simulink model "Controller"  (R2022b)
settings: Solver=FixedStepDiscrete  StartTime=0.0  StopTime=10.0  FixedStep=CONTROL_CONST.dt  MaxStep=CONTROL_PARAM.dt  RelTol=1e-3
values from neighbouring files (symbols this model uses):
  CONTROL_PARAM = Simulink.Parameter(CONTROL_PARAM_VALUE)    [controller_init.m]
undefined symbols (not defined in the file or in its folder): actuator_cmd, CONTROL_CONST, DiscIntNeverNeededParam, timestamp
libraries: drivingvehiclecontroller x2, simulink x1, FMT_Model_Lib x1
settings Model: Creator=19114  LastModifiedBy=19114
settings OptimizationCC: DefaultParameterBehavior=Inlined  DefaultUnderspecifiedDataType=single  EnhancedBackFolding=on  PassReuseOutputArgsAs=Individual arguments  ZeroExternalMemoryAtStartup=off  ZeroInternalMemoryAtStartup=off  OptimizeBlockOrder=speed  DifferentSizesBufferReuse=on  OptimizationCustomize=off  EfficientTunableParamExpr=on
settings DebuggingCC: ParameterTunabilityLossMsg=error  UnconnectedInputMsg=warning  UnconnectedOutputMsg=warning  UnconnectedLineMsg=warning
settings HardwareCC: ProdBitPerPointer=32  ProdBitPerSizeT=32  ProdBitPerPtrDiffT=32  ProdLargestAtomicInteger=Long  ProdLargestAtomicFloat=Double  ProdWordSize=32  ProdHWDeviceType=ARM Compatible->ARM Cortex-M
settings ModelReferenceCC: EnableRefExpFcnMdlSchedulingChecks=on
settings RTWCC: Description=Embedded Coder  SystemTargetFile=ert.tlc  TemplateMakefile=ert_default_tmf  DLArmComputeVersion=19.05
settings CodeAppCC: ForceParamTrailComments=on  IgnoreCustomStorageClasses=off  OperatorAnnotations=on  SimulinkDataObjDesc=on  SFDataObjDesc=on  InsertBlockDesc=on
settings ERTTargetCC: TargetLangStandard=C99 (ISO)  CodeReplacementLibrary=STM32 DSP LIB  GenerateSampleERTMain=on  SupportNonFinite=off  SupportVariableSizeSignals=on  InlinedParameterPlacement=NonHierarchical  ERTCustomFileTemplate=example_file_process.tlc

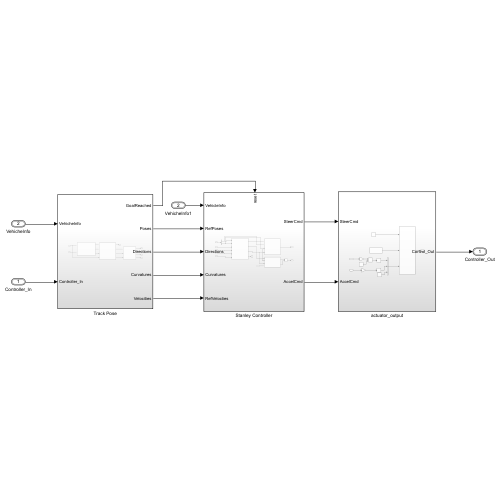
[thumbnail: Simulink's stored preview of the top-level diagram]
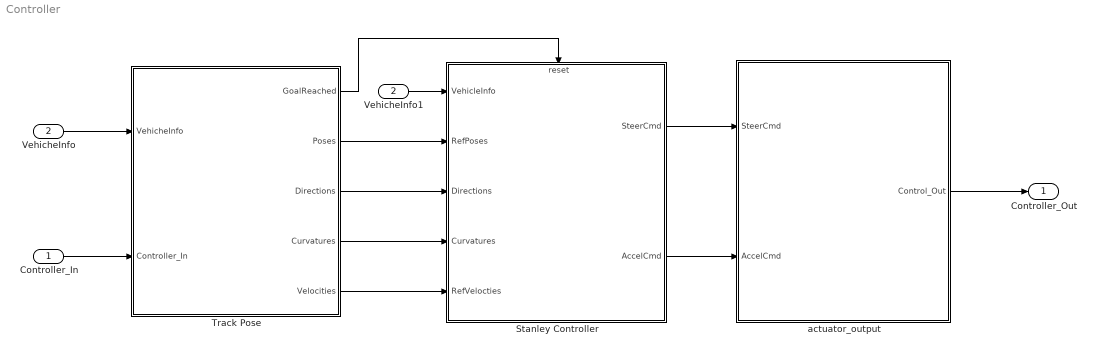
== system Controller ==
  Controller_In : Inport  OutDataTypeStr=Bus: Controller_In_Bus
  VehicheInfo : Inport  Port=2  OutDataTypeStr=Bus: VehicheInfo_Bus
  Stanley Controller : Subsystem
      settings: PortSchema="{\"entries\":[{\"content\":{\"sides\":[{\"content\":{\"connectorIds\":[\"In1\",\"In2\",\"In3\",\"In4\",\"In5\"]},\"type\":\"ConnectorPlacement.EquallySpacedRectSide\",\"uuid\":\"91070305-29de-4808-baf6-dcc08d2076f6\"},{\"content\":{\"connectorIds\":[\"Out1\",\"Out2\"],\"side\":\"RIGHT\"},\"type\":\"ConnectorPlacement.EquallySpacedRectSide\",\"uuid\":\"ca97d8aa-66c0-44c7-8bf0-9bd2dfebf383\"},{\"content\":{\"connectorIds\":[\"In6\"],\"side\":\"TOP\"},\"type\":\"ConnectorPlacement.EquallySpacedRectSide\",\"uuid\":\"0b1186ad-a9e2-4df0-8133-481be95c9fc4\"},{\"content\":{\"connectorIds\":[],\"side\":\"BOTTOM\"},\"type\":\"ConnectorPlacement.EquallySpacedRectSide\",\"uuid\":\"ab154ce3-e196-4faf-b6b9-1e885093f3b6\"}]},\"type\":\"ConnectorPlacement.EquallySpacedConnector\",\"uuid\":\"3fcf1bb3-7915-4a36-93c3-601b19fd5f1b\"}],\"packageUris\":[\"http://schema.mathworks.com/mf0/Connector/R2020b\"],\"version\":\"1.0\"}"
  Track Pose : Subsystem
  VehicheInfo1 : InportShadow  Port=2  OutDataTypeStr=Bus: VehicheInfo_Bus
  actuator_output : Subsystem
  Controller_Out : Outport  OutDataTypeStr=Bus: Controller_Out_Bus
  wires:
  Stanley Controller/1(SteerCmd) -> actuator_output/1(SteerCmd)
  Stanley Controller/2(AccelCmd) -> actuator_output/2(AccelCmd)
  actuator_output/1(Control_Out) -> Controller_Out/1
  VehicheInfo/1 -> Track Pose/1(VehicheInfo)
  Controller_In/1 -> Track Pose/2(Controller_In)
  Track Pose/1(GoalReached) -> Stanley Controller/6(reset)
  Track Pose/2(Poses) -> Stanley Controller/2(RefPoses)
  Track Pose/3(Directions) -> Stanley Controller/3(Directions)
  Track Pose/4(Curvatures) -> Stanley Controller/4(Curvatures)
  Track Pose/5(Velocities) -> Stanley Controller/5(RefVelocties)
  VehicheInfo1/1 -> Stanley Controller/1(VehicleInfo)

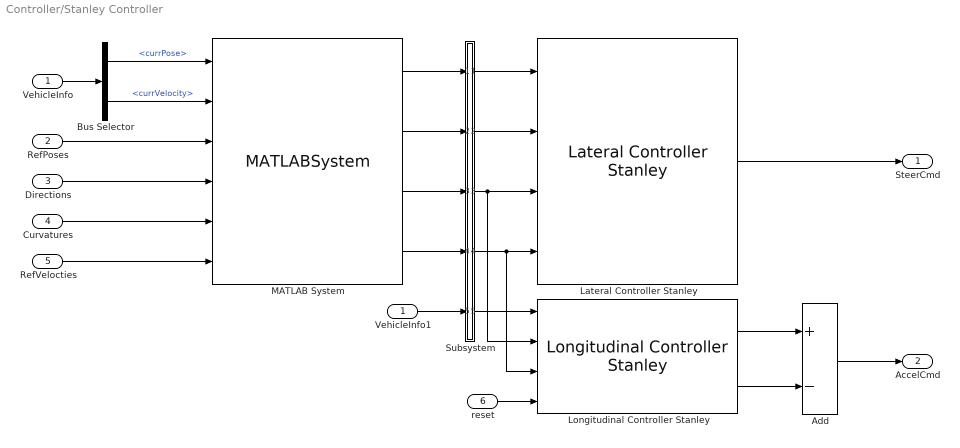
== system Controller/Stanley Controller ==
  VehicleInfo : Inport
  RefPoses : Inport  Port=2
  Directions : Inport  Port=3
  Curvatures : Inport  Port=4
  RefVelocties : Inport  Port=5
  reset : Inport  Port=6
  Add : Sum  Inputs=+-
  Bus Selector : BusSelector  OutputSignals=currPose,currVelocity
  Lateral Controller Stanley : drivingvehiclecontroller/Lateral Controller Stanley  ModelType=Kinematic bicycle model  PositionGainF=2  PositionGainR=2.5  YawRateGain=0.25  DelayGain=0.2  VehicleMass=5  Lf=1.2  Lr=1.6  TireStiffness=19e3  Wheelbase=0.3  MaxSteeringAngle=30
  Longitudinal Controller Stanley : drivingvehiclecontroller/Longitudinal Controller Stanley  Kp=CONTROL_PARAM.KP  Ki=CONTROL_PARAM.KI  SampleTime=CONTROL_CONST.dt  MaxAcceleration=20  MaxDeceleration=20
  MATLAB System : MATLABSystem  System=HelperPathAnalyzer  Wheelbase=2.8  HasResetOutput=off  SimulateUsing=Code generation
      mask Type: HelperPathAnalyzer
      mask Display:
      | disp(['Helper' char(10) 'Path' char(10) 'Analyzer']);
      | port_label('input',1,'CurrPose');
      | port_label('input',2,'CurrVelocity');
      | port_label('input',3,'RefPoses');
      | port_label('input',4,'Directions');
      | port_label('input',5,'Curvatures');
      | port_label('input',6,'RefVelocities');
      | port_label('output',1,'RefPose');
      | port_label('output',2,'RefVelocity');
      | port_label('output',3,'Direction');
      | port_label('output',4,'Curvature');
  Subsystem : Subsystem
  VehicleInfo1 : InportShadow
  SteerCmd : Outport
  AccelCmd : Outport  Port=2
  wires:
  VehicleInfo/1 -> Bus Selector/1
  Bus Selector/2 -> MATLAB System/2  "<currVelocity>"
  Bus Selector/1 -> MATLAB System/1  "<currPose>"
  RefPoses/1 -> MATLAB System/3
  Directions/1 -> MATLAB System/4
  Curvatures/1 -> MATLAB System/5
  RefVelocties/1 -> MATLAB System/6
  Lateral Controller Stanley/1 -> SteerCmd/1
  Longitudinal Controller Stanley/1 -> Add/1
  Longitudinal Controller Stanley/2 -> Add/2
  Add/1 -> AccelCmd/1
  reset/1 -> Longitudinal Controller Stanley/4
  MATLAB System/1 -> Subsystem/1(RefPose)
  MATLAB System/2 -> Subsystem/2(RefVelocity)
  MATLAB System/3 -> Subsystem/3(Direction)
  MATLAB System/4 -> Subsystem/4(Curvature)
  VehicleInfo1/1 -> Subsystem/5(VehicleInfo)
  Subsystem/1(RefPose1) -> Lateral Controller Stanley/1
  Subsystem/2(CurrPose) -> Lateral Controller Stanley/2
  Subsystem/3(CurrVelocity) -> Longitudinal Controller Stanley/2, Lateral Controller Stanley/3
  Subsystem/4(Direction1) -> Longitudinal Controller Stanley/3, Lateral Controller Stanley/4
  Subsystem/5(RefVelocity1) -> Longitudinal Controller Stanley/1

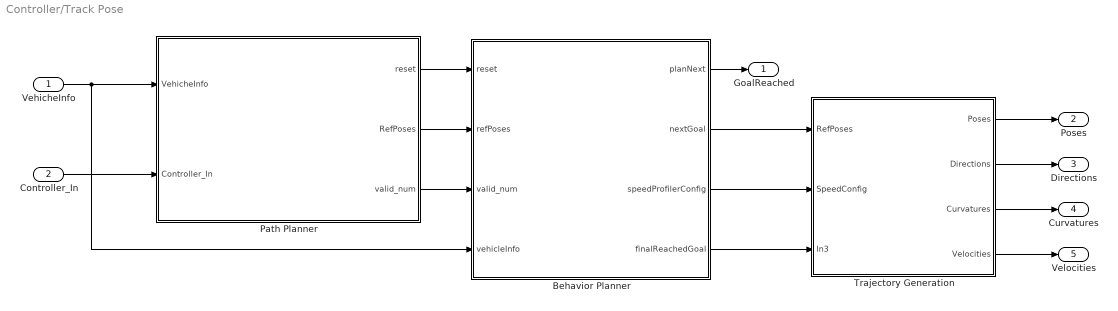
== system Controller/Track Pose ==
  VehicheInfo : Inport
  Controller_In : Inport  Port=2
  Behavior Planner : MATLAB Function  TreatAsAtomicUnit=on
  Path Planner : Subsystem
  Trajectory Generation : Subsystem
  GoalReached : Outport
  Poses : Outport  Port=2
  Directions : Outport  Port=3
  Curvatures : Outport  Port=4
  Velocities : Outport  Port=5
  wires:
  Behavior Planner/4(finalReachedGoal) -> Trajectory Generation/3(In3)
  Behavior Planner/3(speedProfilerConfig) -> Trajectory Generation/2(SpeedConfig)
  Trajectory Generation/2(Directions) -> Directions/1
  Path Planner/1(reset) -> Behavior Planner/1(reset)
  Path Planner/3(valid_num) -> Behavior Planner/3(valid_num)
  Behavior Planner/2(nextGoal) -> Trajectory Generation/1(RefPoses)
  Path Planner/2(RefPoses) -> Behavior Planner/2(refPoses)
  Trajectory Generation/3(Curvatures) -> Curvatures/1
  Behavior Planner/1(planNext) -> GoalReached/1
  VehicheInfo/1 -> Behavior Planner/4(vehicleInfo), Path Planner/1(VehicheInfo)
  Trajectory Generation/4(Velocities) -> Velocities/1
  Trajectory Generation/1(Poses) -> Poses/1
  Controller_In/1 -> Path Planner/2(Controller_In)

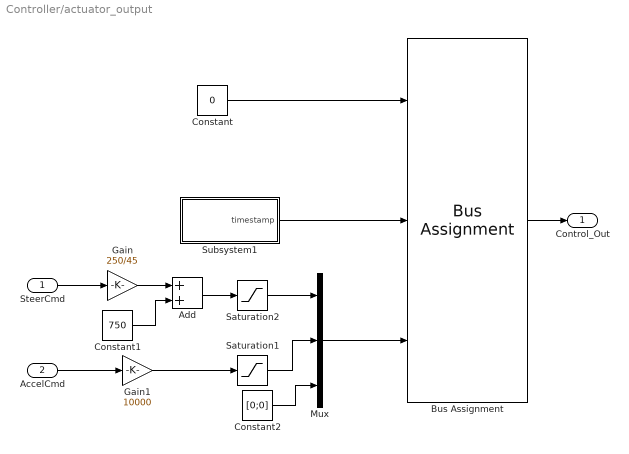
== system Controller/actuator_output ==
  SteerCmd : Inport
  AccelCmd : Inport  Port=2
  Add : Sum
  Bus Assignment : BusAssignment  AssignedSignals=timestamp,actuator_cmd
  Constant : Constant  Value=0  OutDataTypeStr=Bus: Controller_Out_Bus
  Constant1 : Constant  Value=750
  Constant2 : Constant  Value=[0;0]  OutDataTypeStr=int16
  Gain : Gain  Gain=250/45
  Gain1 : Gain  Gain=10000
  Mux : Mux  Inputs=3
  Saturation1 : Saturate  UpperLimit=10000  LowerLimit=-10000  OutDataTypeStr=int16
  Saturation2 : Saturate  UpperLimit=1250  LowerLimit=250  OutDataTypeStr=int16
  Subsystem1 : Subsystem
  Control_Out : Outport
  wires:
  Saturation2/1 -> Mux/1
  SteerCmd/1 -> Gain/1
  Saturation1/1 -> Mux/2
  Gain1/1 -> Saturation1/1
  Subsystem1/1(timestamp) -> Bus Assignment/2
  Mux/1 -> Bus Assignment/3
  Constant2/1 -> Mux/3
  Constant1/1 -> Add/2
  Add/1 -> Saturation2/1
  Constant/1 -> Bus Assignment/1
  Gain/1 -> Add/1
  Bus Assignment/1 -> Control_Out/1
  AccelCmd/1 -> Gain1/1

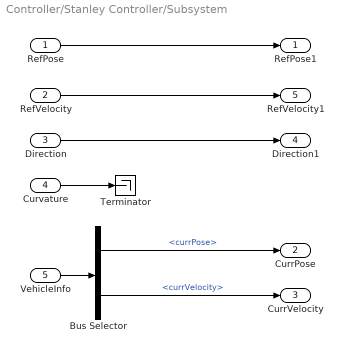
== system Controller/Stanley Controller/Subsystem ==
  RefPose : Inport
  RefVelocity : Inport  Port=2
  Direction : Inport  Port=3
  Curvature : Inport  Port=4
  VehicleInfo : Inport  Port=5
  Bus Selector : BusSelector  OutputSignals=currPose,currVelocity
  Terminator : Terminator
  RefPose1 : Outport
  CurrPose : Outport  Port=2
  CurrVelocity : Outport  Port=3
  Direction1 : Outport  Port=4
  RefVelocity1 : Outport  Port=5
  wires:
  RefPose/1 -> RefPose1/1
  VehicleInfo/1 -> Bus Selector/1
  Bus Selector/1 -> CurrPose/1  "<currPose>"
  Bus Selector/2 -> CurrVelocity/1  "<currVelocity>"
  Direction/1 -> Direction1/1
  RefVelocity/1 -> RefVelocity1/1
  Curvature/1 -> Terminator/1

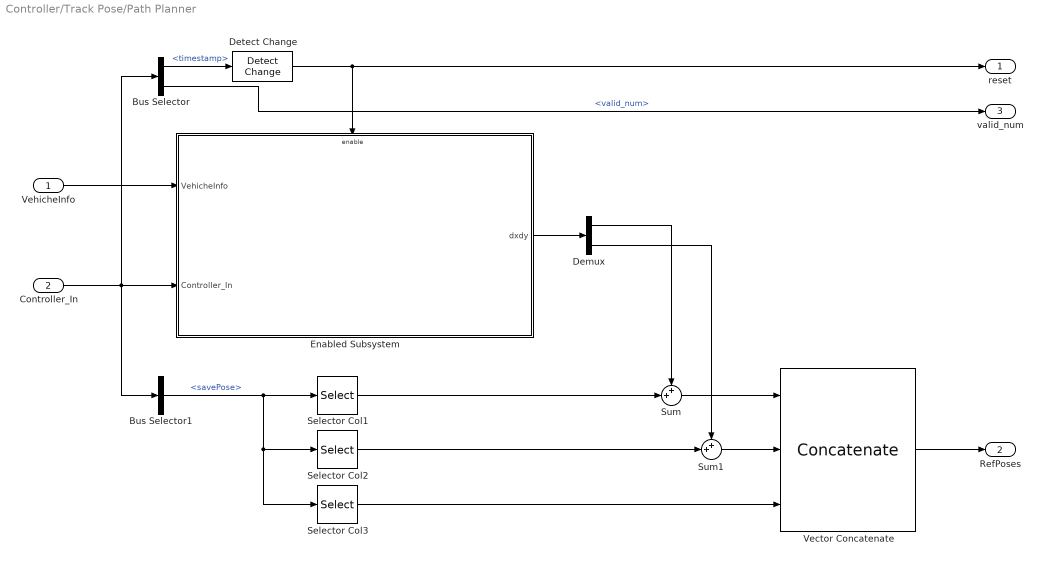
== system Controller/Track Pose/Path Planner ==
  VehicheInfo : Inport
  Controller_In : Inport  Port=2
  Bus Selector : BusSelector  OutputSignals=timestamp,valid_num
  Bus Selector1 : BusSelector  OutputSignals=savePose
  Demux : Demux  Outputs=2
  Detect Change : simulink/Logic and Bit Operations/Detect Change  vinit=0  OutDataTypeStr=boolean
  Enabled Subsystem : Subsystem  TreatAsAtomicUnit=on
  Selector Col1 : Selector  NumberOfDimensions=2  InputPortWidth=3  IndexOptions=Select all,Index vector (dialog)  Indices=[1 3],1  OutputSizes=1,1
  Selector Col2 : Selector  NumberOfDimensions=2  InputPortWidth=3  IndexOptions=Select all,Index vector (dialog)  Indices=[1 3],2  OutputSizes=1,1
  Selector Col3 : Selector  NumberOfDimensions=2  InputPortWidth=3  IndexOptions=Select all,Index vector (dialog)  Indices=[1 3],3  OutputSizes=1,1
  Sum : Sum  Inputs=++|
  Sum1 : Sum  Inputs=++|
  Vector Concatenate : Concatenate  NumInputs=3  Mode=Multidimensional array  ConcatenateDimension=2
  reset : Outport
  RefPoses : Outport  Port=2
  valid_num : Outport  Port=3
  wires:
  Bus Selector/1 -> Detect Change/1  "<timestamp>"
  Bus Selector1/1 -> Selector Col3/1, Selector Col2/1, Selector Col1/1  "<savePose>"
  Selector Col1/1 -> Sum/2
  Demux/2 -> Sum1/1
  Enabled Subsystem/1(dxdy) -> Demux/1
  Detect Change/1 -> reset/1, Enabled Subsystem/Enable
  Sum/1 -> Vector Concatenate/1
  Selector Col2/1 -> Sum1/2
  Demux/1 -> Sum/1
  Sum1/1 -> Vector Concatenate/2
  Controller_In/1 -> Bus Selector1/1, Bus Selector/1, Enabled Subsystem/2(Controller_In)
  Selector Col3/1 -> Vector Concatenate/3
  VehicheInfo/1 -> Enabled Subsystem/1(VehicheInfo)
  Vector Concatenate/1 -> RefPoses/1
  Bus Selector/2 -> valid_num/1  "<valid_num>"

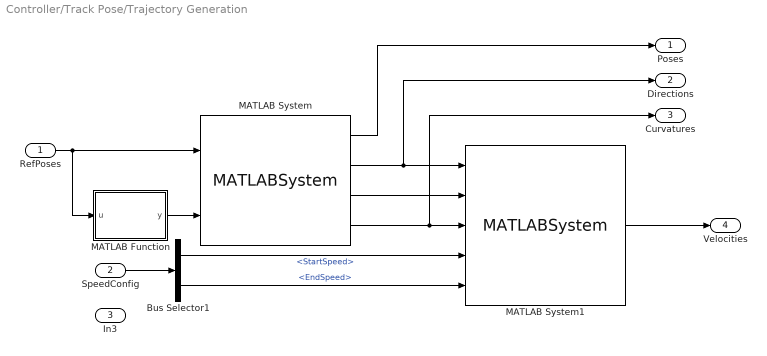
== system Controller/Track Pose/Trajectory Generation ==
  RefPoses : Inport
  SpeedConfig : Inport  Port=2
  In3 : Inport  Port=3
  Bus Selector1 : BusSelector  OutputSignals=StartSpeed,EndSpeed
  MATLAB Function : MATLAB Function  TreatAsAtomicUnit=on
  MATLAB System : MATLABSystem  System=PathSmootherSpline  NumSmoothPoses=50  MinSeparation=1e-3  SampleTime=-1  ShowOptionalOutports=on  SimulateUsing=Code generation
      mask Type: PathSmootherSpline
      mask Display:
      | disp(['Path' char(10) 'Smoother' char(10) 'Spline']);
      | port_label('input',1,'RefPoses');
      | port_label('input',2,'RefDirections');
      | port_label('output',1,'Poses');
      | port_label('output',2,'Directions');
      | port_label('output',3,'CumLengths');
      | port_label('output',4,'Curvatures');
  MATLAB System1 : MATLABSystem  System=VelocityProfiler  MaxLongitudinalAccel=20  MaxLongitudinalDecel=20  MaxSpeed=20  MaxLongitudinalJerk=10  MaxLateralAccel=20  ShowOptionalOutport=off  SampleTime=-1  SimulateUsing=Code generation
      mask Type: VelocityProfiler
      mask Display:
      | disp(['Velocity' char(10) 'Profiler']);
      | port_label('input',1,'Directions');
      | port_label('input',2,'CumLengths');
      | port_label('input',3,'Curvatures');
      | port_label('input',4,'StartVelocity');
      | port_label('input',5,'EndVelocity');
      | port_label('output',1,'Velocities');
  Poses : Outport  VectorParamsAs1DForOutWhenUnconnected=off
  Directions : Outport  Port=2  VectorParamsAs1DForOutWhenUnconnected=off
  Curvatures : Outport  Port=3  VectorParamsAs1DForOutWhenUnconnected=off
  Velocities : Outport  Port=4  VectorParamsAs1DForOutWhenUnconnected=off
  wires:
  MATLAB System1/1 -> Velocities/1
  MATLAB System/2 -> MATLAB System1/1, Directions/1
  MATLAB System/4 -> MATLAB System1/3, Curvatures/1
  Bus Selector1/2 -> MATLAB System1/5  "<EndSpeed>"
  RefPoses/1 -> MATLAB System/1, MATLAB Function/1(u)
  Bus Selector1/1 -> MATLAB System1/4  "<StartSpeed>"
  MATLAB System/3 -> MATLAB System1/2
  MATLAB System/1 -> Poses/1
  MATLAB Function/1(y) -> MATLAB System/2
  SpeedConfig/1 -> Bus Selector1/1

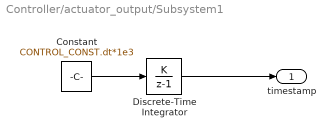
== system Controller/actuator_output/Subsystem1 ==
  Constant : Constant  Value=CONTROL_CONST.dt*1e3  OutDataTypeStr=uint32
  Discrete-Time Integrator : DiscreteIntegrator  IntegratorMethod=Accumulation: Forward Euler  gainval=1  SampleTime=-1  ICPrevOutput=DiscIntNeverNeededParam  ICPrevScaledInput=DiscIntNeverNeededParam
  timestamp : Outport
  wires:
  Constant/1 -> Discrete-Time Integrator/1
  Discrete-Time Integrator/1 -> timestamp/1

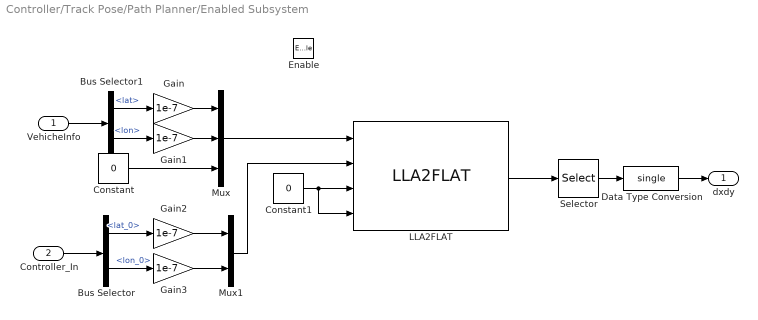
== system Controller/Track Pose/Path Planner/Enabled Subsystem ==
  VehicheInfo : Inport
  Controller_In : Inport  Port=2
  Enable : EnablePort
  Bus Selector : BusSelector  OutputSignals=lat_0,lon_0
  Bus Selector1 : BusSelector  OutputSignals=lat,lon
  Constant : Constant  Value=0  OutDataTypeStr=double
  Constant1 : Constant  Value=0  OutDataTypeStr=double
  Data Type Conversion : DataTypeConversion  OutDataTypeStr=single  SaturateOnIntegerOverflow=off  RndMeth=Floor
  Gain{,1..3} (4 alike) : Gain  Gain=1e-7  OutDataTypeStr=double
  LLA2FLAT : FMT_Model_Lib/Transformation/LLA2FLAT
      settings: SourceProductName=FMT Toolbox
  Mux : Mux  Inputs=3
  Mux1 : Mux  Inputs=2
  Selector : Selector  InputPortWidth=3  IndexOptions=Index vector (dialog)  Indices=[1 2]  OutputSizes=1
  dxdy : Outport
  wires:
  Mux1/1 -> LLA2FLAT/2
  Constant/1 -> Mux/3
  Mux/1 -> LLA2FLAT/1
  Constant1/1 -> LLA2FLAT/4, LLA2FLAT/3
  Controller_In/1 -> Bus Selector/1
  VehicheInfo/1 -> Bus Selector1/1
  LLA2FLAT/1 -> Selector/1
  Gain/1 -> Mux/1
  Bus Selector1/1 -> Gain/1  "<lat>"
  Bus Selector1/2 -> Gain1/1  "<lon>"
  Gain1/1 -> Mux/2
  Bus Selector/1 -> Gain2/1  "<lat_0>"
  Bus Selector/2 -> Gain3/1  "<lon_0>"
  Gain3/1 -> Mux1/2
  Gain2/1 -> Mux1/1
  Selector/1 -> Data Type Conversion/1
  Data Type Conversion/1 -> dxdy/1

== matlab function Controller/Track Pose/Behavior Planner ==
  data: reset input; planNext output; refPoses input; valid_num input; vehicleInfo input Bus: VehicheInfo_Bus; nextGoal output; speedProfilerConfig output Bus: SpeedConfig_Bus; finalReachedGoal output
function [planNext, nextGoal, speedProfilerConfig, finalReachedGoal] = ...
    behaviorPlanning(reset, refPoses, valid_num, vehicleInfo)

%behaviorPlanning generate navigation tasks and configurations for the 
%   Motion Planner block and the Trajectory Generator block.
nextGoal   = coder.nullcopy(zeros(2, 3, 'single')); %#ok<*NASGU>
planNext   = coder.nullcopy(logical(0));  %#ok<*LOGL>

persistent goalIndex finalReached endSpeed
persistent nextGoalPose speedConfig

if isempty(goalIndex) || reset > 0
    % Initialize pose and speed
    finalReached = logical(0);
    endSpeed  = single(1);
    goalIndex = 1;
    nextGoalPose = [vehicleInfo.currPose ;refPoses(goalIndex,:)];
    speedConfig.StartSpeed  = vehicleInfo.currVelocity;
    speedConfig.EndSpeed    = endSpeed;
    goalIndex = goalIndex + 1;
end

planNext = logical(0);
if ~finalReached
    % Plan a new path when reaching the goal
    if helperGoalChecker(nextGoalPose(end, :), vehicleInfo.currPose, vehicleInfo.currVelocity, speedConfig.EndSpeed, vehicleInfo.direction)
        if goalIndex <= valid_num
            nextGoalPose = [refPoses(goalIndex,:) ;refPoses(goalIndex+1,:)];
            speedConfig.StartSpeed  = vehicleInfo.currVelocity;
            speedConfig.EndSpeed    = endSpeed;
            goalIndex = goalIndex + 1;
            planNext = logical(1);
        else
            % reach the last goal, clear setting pose and velocity.
            nextGoalPose(:, :) = single(0);
            speedConfig.StartSpeed = single(0);
            speedConfig.EndSpeed = single(0);
            finalReached       = logical(1);
        end
    end
end
    
finalReachedGoal    = finalReached;
nextGoal            = nextGoalPose;
speedProfilerConfig = speedConfig;

end

== matlab function Controller/Track Pose/Trajectory Generation/MATLAB Function ==
  data: u input; y output
function y = fcn(u)

y = ones([size(u, 1), 1], 'like',u);
